simulink model "States6_2018a"  (R2018a)
settings: Solver=FixedStepDiscrete  StartTime=0.0  StopTime=0.1  FixedStep=0.1  RelTol=1e-3  EnableMultiTasking=on
settings Model: Creator=bzhan  LastModifiedBy=bzhan
settings SolverCC: AutoInsertRateTranBlk=on
settings DataIOCC: LimitDataPoints=on  ReturnWorkspaceOutputs=on
settings OptimizationCC: LifeSpan=inf
settings DebuggingCC: AllowSymbolicDim=off  SFUnexpectedBacktrackingDiag=warning  SFNoUnconditionalDefaultTransitionDiag=warning  SFExecutionAtInitializationDiag=none
settings CodeAppCC: StateflowObjectComments=on
settings GRTTargetCC: TargetLangStandard=C89/C90 (ANSI)
settings ConfigComp: CovMetricSettings=dw  CovHtmlReporting=on  CovSaveCumulativeToWorkspaceVar=on  CovSaveSingleToWorkspaceVar=on  CovShowResultsExplorer=off  CovExternalEMLEnable=off  CovSFcnEnable=off

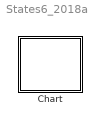
== system States6_2018a ==
  Chart : Stateflow chart  TreatAsAtomicUnit=on

== stateflow chart States6_2018a/Chart ==
  settings: updateMethod=DISCRETE  sampleTime=0.1
  state A [parallel]
    en: f("enA")
    settings: executionOrder=1
    state A1 [parallel]
      en: f("enA1")
      settings: executionOrder=1
    state A2 [parallel]
      en: f("enA2")
      settings: executionOrder=2
  state B [parallel]
    en: f("enB")
    settings: executionOrder=2
    state B1 [parallel]
      en: f("enB1")
      settings: executionOrder=1
    state B2 [parallel]
      en: f("enB2")
      settings: executionOrder=2
  data: s function_input
  function f(s):
    | function f(s)
    |   fprintf(s+"\n");
